simulink model "segmentation_exercise"  (R2021a)
settings: Solver=FixedStepAuto  StartTime=0.0  StopTime=100  RelTol=1e-3
libraries: visionstatistics x1, simulink x1, visiontextngfix x1, visiongeotforms x1, visionsources x1
settings Model: Creator=lipingw  LastModifiedBy=mmordeka
settings SolverCC: AlgebraicLoopSolver=TrustRegion
settings DebuggingCC: SFMachineParentedDataDiag=warning

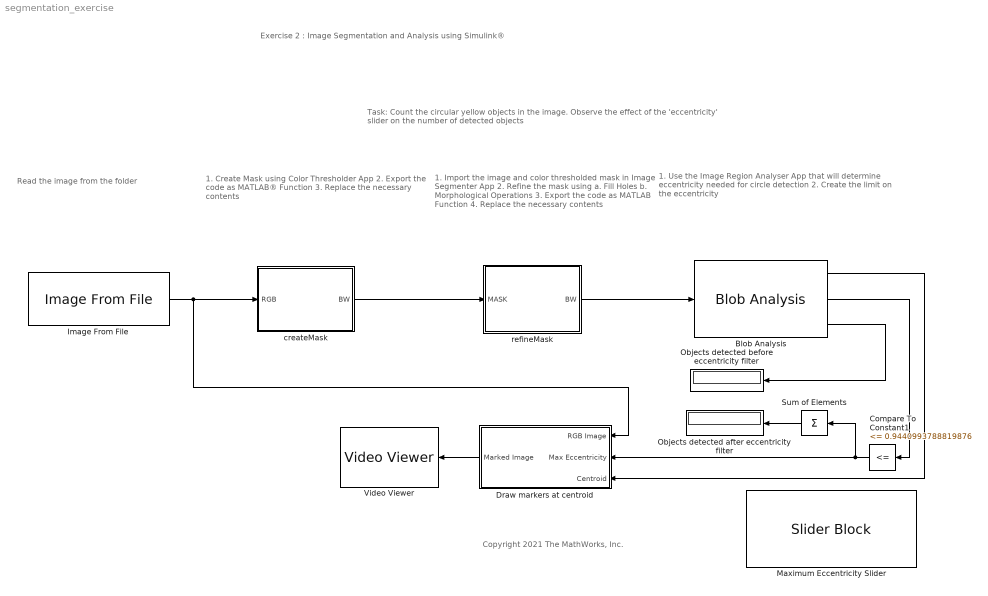
== system segmentation_exercise ==
  note: Copyright 2021 The MathWorks, Inc.
  note: Exercise 2 : Image Segmentation and Analysis
      | using Simulink®
  note: 1. Use the Image Region Analyser App
      | that will determine eccentricity needed for circle
      | detection
      | 2. Create the limit on the eccentricity
  note: 1. Import the image and color thresholded
      | mask in Image Segmenter App
      | 2. Refine the mask using
      | 	a. Fill Holes
      | 	b. Morphological Operations
      | 3. Export the code as MATLAB Function
      | 4. Replace the necessary contents
  note: 1. Create Mask using Color Thresholder App
      | 2. Export the code as MATLAB® Function
      | 3. Replace the necessary contents
  note: Read the image from the folder
  note: Task: Count the circular yellow objects in the image. Observe the effect of the 'eccentricity' slider on the number of detected objects
  Blob Analysis : visionstatistics/Blob Analysis  Tag=vipblks_row_conv  area=off  centroid=on  bBox=off  majorAxis=off  minorAxis=off  angle=off  eccentricity=on  equivDiameterSq=off  extent=off  perimeter=off  outDT=double  conn=8  isLabel=off  maxBlobs=50  warnIfNumBlobsExceeded=on  isCount=on  useMinArea=off  minArea=0  useMaxArea=off  maxArea=intmax('uint32')  excludeBorderBlob=off  isOutVarDim=on  isFill=on  fillValues=0  roundingMode=Floor  overflowMode=off  prodOutputMode=Binary point scaling  prodOutputWordLength=32  prodOutputFracLength=16  accumMode=Binary point scaling  accumWordLength=32  accumFracLength=0  outputMode=Binary point scaling  outputWordLength=32  outputFracLength=16  firstCoeffMode=Binary point scaling  firstCoeffWordLength=16  firstCoeffFracLength=14  secondCoeffMode=Binary point scaling  secondCoeffWordLength=32  secondCoeffFracLength=16
  Compare To Constant1 : simulink/Logic and Bit Operations/Compare To Constant  relop=<=  const=0.9440993788819876  OutDataTypeStr=boolean
  Draw markers at centroid : Subsystem
  Image From File : visionsources/Image From File  Tag=vipblks_nd  FileName=yellowObjects.jpg  Ts=Inf  imagePorts=One multidimensional signal  OutPortLabels=R|G|B  ImageDataType=Inherit from input image  sdImageDataType=uint(8)  Signed=on  WordLength=16  FractionLengthMode=User-defined  FractionLength=15
  Maximum Eccentricity Slider : SliderBlock  ScaleMax=1
  Objects detected after eccentricity filter : Display
  Objects detected before eccentricity filter : Display
  Sum of Elements : Sum  Inputs=+
  Video Viewer : VideoViewer  FigPos=[1158 652 765 544]
  createMask : MATLAB Function  TreatAsAtomicUnit=on
  refineMask : MATLAB Function  TreatAsAtomicUnit=on
  wires:
  refineMask/1(BW) -> Blob Analysis/1
  createMask/1(BW) -> refineMask/1(MASK)
  Blob Analysis/2 -> Compare To Constant1/1
  Blob Analysis/3 -> Objects detected before eccentricity filter/1
  Compare To Constant1/1 -> Sum of Elements/1, Draw markers at centroid/2(Max Eccentricity)
  Draw markers at centroid/1(Marked Image) -> Video Viewer/1
  Image From File/1 -> Draw markers at centroid/1(RGB Image), createMask/1(RGB)
  Blob Analysis/1 -> Draw markers at centroid/3(Centroid)
  Sum of Elements/1 -> Objects detected after eccentricity filter/1

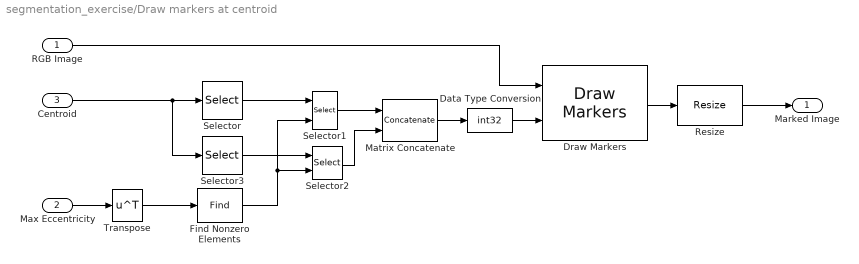
== system segmentation_exercise/Draw markers at centroid ==
  RGB Image : Inport
  Max Eccentricity : Inport  Port=2
  Centroid : Inport  Port=3
  Data Type Conversion : DataTypeConversion  OutDataTypeStr=int32
  Draw Markers : visiontextngfix/Draw Markers  shape=X-mark  size=5  fill=on  fillClrSource=Specify via dialog  display=Black  intensity=200  color=[200 255 100]  opacity=0.6  viewport=Entire image  antialiasing=off  inType=Obsolete  imagePorts=One multidimensional signal  roundingMode=Floor  overflowMode=off  memoryMode=Specify word length  memoryWordLength=16  memoryFracLength=15  prodOutputMode=Binary point scaling  prodOutputWordLength=32  prodOutputFracLength=14
      settings: SourceProductBaseCode=VP
  Find Nonzero Elements : Find  NumberOfInputDimensions=3  IndexMode=Zero-based
  Matrix Concatenate : Concatenate  Mode=Multidimensional array  ConcatenateDimension=2
  Resize : visiongeotforms/Resize  specify=Output size as a percentage of input size  rfactor=[75 75]  outCols=25  outRows=25  outRowsCols=[25 35]  interp_method=Bilinear  antialias=on  useROI=off  roiFlag=off  roundingMode=Nearest  overflowMode=on  prodOutputMode=Binary point scaling  prodOutputWordLength=32  prodOutputFracLength=10
      settings: SourceProductBaseCode=VP
  Selector : Selector  NumberOfDimensions=2  InputPortWidth=3  IndexOptions=Select all,Index vector (dialog)  Indices=[1],[1]  OutputSizes=1,1
  Selector1 : Selector  IndexMode=Zero-based  InputPortWidth=50  IndexOptions=Index vector (port)  Indices=[1 3]  OutputSizes=1
  Selector2 : Selector  IndexMode=Zero-based  InputPortWidth=50  IndexOptions=Index vector (port)  Indices=[1 3]  OutputSizes=1
  Selector3 : Selector  NumberOfDimensions=2  InputPortWidth=3  IndexOptions=Select all,Index vector (dialog)  Indices=[2],[2]  OutputSizes=1,1
  Transpose : Math  Operator=transpose  SaturateOnIntegerOverflow=on
  Marked Image : Outport
  wires:
  Selector2/1 -> Matrix Concatenate/2
  Selector1/1 -> Matrix Concatenate/1
  Transpose/1 -> Find Nonzero Elements/1
  Max Eccentricity/1 -> Transpose/1
  Selector3/1 -> Selector2/1
  Selector/1 -> Selector1/1
  Find Nonzero Elements/1 -> Selector2/2, Selector1/2
  Centroid/1 -> Selector/1, Selector3/1
  RGB Image/1 -> Draw Markers/1
  Matrix Concatenate/1 -> Data Type Conversion/1
  Draw Markers/1 -> Resize/1
  Resize/1 -> Marked Image/1
  Data Type Conversion/1 -> Draw Markers/2

== matlab function segmentation_exercise/createMask ==
  data: RGB input; BW output
function BW  = createMask(RGB)

I = RGB;

%Add the auto generated MATLAB Function thresholds 
% from the Color Thresholder App

% Create mask based on chosen histogram thresholds
sliderBW = (I(:,:,1) >= channel1Min ) & (I(:,:,1) <= channel1Max) & ...
    (I(:,:,2) >= channel2Min ) & (I(:,:,2) <= channel2Max) & ...
    (I(:,:,3) >= channel3Min ) & (I(:,:,3) <= channel3Max);
BW = sliderBW;

end

== matlab function segmentation_exercise/refineMask ==
  data: MASK input; BW output
function BW = refineMask(MASK)
% Add the auto-generated code from Image Segmenter App to
% 1. Fill Holes 
% 2. Perform morphological operations
